simulink model "rotacionalSimulink"  (R2023b)
settings: Solver=VariableStepAuto  StartTime=0.0  StopTime=10.0  RelTol=1e-3
values from neighbouring files (symbols this model uses):
  k = 100    [PRCT4.m]    (also in PRCT4S.m)
  m = 10    [PRCT4.m]    (also in PRCT4S.m)
settings Model: Creator=ZBOOK 15 G7

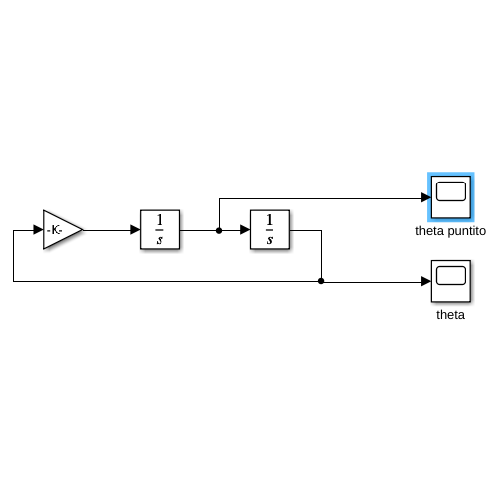
[thumbnail: Simulink's stored preview of the top-level diagram]
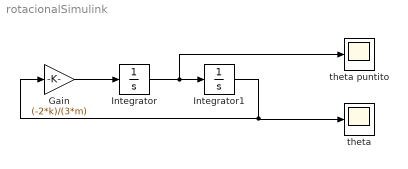
== system rotacionalSimulink ==
  Gain : Gain  Gain=(-2*k)/(3*m)
  Integrator : Integrator  InitialCondition=2
  Integrator1 : Integrator
  theta : Scope
  theta puntito : Scope
  wires:
  Integrator/1 -> theta puntito/1, Integrator1/1
  Gain/1 -> Integrator/1
  Integrator1/1 -> Gain/1, theta/1
